simulink model "ekf_drone_3d"  (R2026a)
settings: Solver=ode4  FixedStep=0.01
libraries: simulink x1
settings Model: Creator=jaivi  LastModifiedBy=jaivi

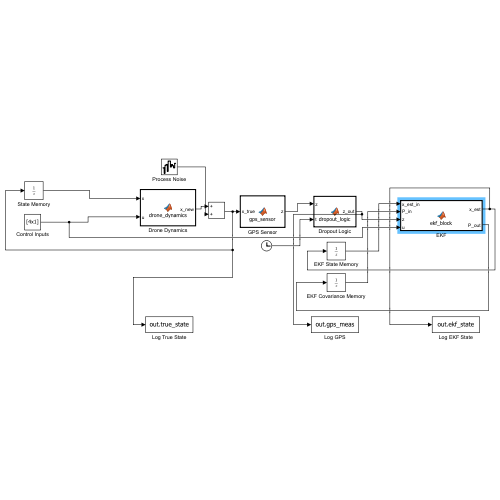
[thumbnail: Simulink's stored preview of the top-level diagram]
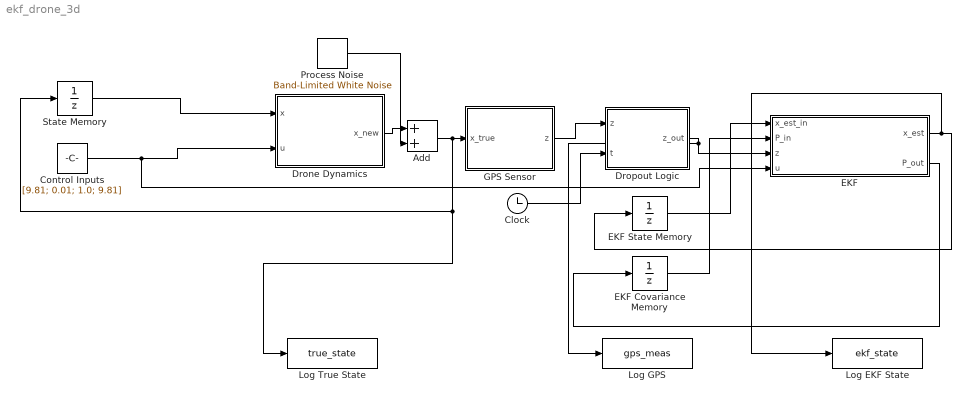
== system ekf_drone_3d ==
  Add : Sum
  Clock : Clock
  Control Inputs : Constant  Value=[9.81; 0.01; 1.0; 9.81]  OutDataTypeStr=double
  Drone Dynamics : MATLAB Function  TreatAsAtomicUnit=on
  Dropout Logic : MATLAB Function  TreatAsAtomicUnit=on
  EKF : MATLAB Function  TreatAsAtomicUnit=on
  EKF Covariance Memory : UnitDelay  InitialCondition=0.1*ones(64,1)  SampleTime=0.01
  EKF State Memory : UnitDelay  InitialCondition=[0; 0; 10; 0; 0; 0; 0; 0]  SampleTime=0.01
  GPS Sensor : MATLAB Function  TreatAsAtomicUnit=on
  Log EKF State : ToWorkspace  VariableName=ekf_state  SampleTime=-1
  Log GPS : ToWorkspace  VariableName=gps_meas  SampleTime=-1
  Log True State : ToWorkspace  VariableName=true_state  SampleTime=-1
  Process Noise : simulink/Sources/Band-Limited White Noise  Cov=[0.001 0.001 0.001 0.002 0.002 0.002 0.0001 0.0001]  Ts=0.01  seed=[23341]
  State Memory : UnitDelay  InitialCondition=[0; 0; 10; 0; 0; 0; 0; 0]  SampleTime=0.01
  wires:
  Control Inputs/1 -> EKF/4(u), Drone Dynamics/2(u)
  State Memory/1 -> Drone Dynamics/1(x)
  GPS Sensor/1(z) -> Dropout Logic/1(z)
  Clock/1 -> Dropout Logic/2(t)
  EKF State Memory/1 -> EKF/1(x_est_in)
  EKF Covariance Memory/1 -> EKF/2(P_in)
  Dropout Logic/1(z_out) -> Log GPS/1, EKF/3(z)
  EKF/1(x_est) -> Log EKF State/1, EKF State Memory/1
  EKF/2(P_out) -> EKF Covariance Memory/1
  Drone Dynamics/1(x_new) -> Add/1
  Process Noise/1 -> Add/2
  Add/1 -> State Memory/1, Log True State/1, GPS Sensor/1(x_true)

== matlab function ekf_drone_3d/GPS Sensor ==
  data: x_true input; z output
function z = gps_sensor(x_true)
% GPS sensor — measures position only with noise
% x_true = [px, py, pz, vx, vy, vz, theta, phi] (8x1)
% z = [px_meas, py_meas, pz_meas] (3x1)

% Extract true position
px = x_true(1);
py = x_true(2);
pz = x_true(3);

% Add Gaussian noise (2m standard deviation)
noise = 2.0 * randn(3,1);

z = [px; py; pz] + noise;

== matlab function ekf_drone_3d/Drone Dynamics ==
  data: x input; u input; x_new output
function x_new = drone_dynamics(x, u)
% 3D drone state transition
% x = [px, py, pz, vx, vy, vz, theta, phi] (8x1)
% u = [T, dt, m, g] inputs and constants

px    = x(1);
py    = x(2);
pz    = x(3);
vx    = x(4);
vy    = x(5);
vz    = x(6);
theta = x(7);
phi   = x(8);

T  = u(1);
dt = u(2);
m  = u(3);
g  = u(4);

% Accelerations
ax =  (T/m) * sin(theta);
ay = -(T/m) * sin(phi) * cos(theta);
az =  (T/m) * cos(phi) * cos(theta) - g;

% Next state
x_new = [
    px + vx*dt;
    py + vy*dt;
    pz + vz*dt;
    vx + ax*dt;
    vy + ay*dt;
    vz + az*dt;
    theta;
    phi
];

== matlab function ekf_drone_3d/Dropout Logic ==
  data: z input; z_out output; t input
function z_out = dropout_logic(z, t)
% Cut GPS signal between t=3s and t=5s
% z = GPS measurement (3x1)
% t = current simulation time

if t >= 3.0 && t <= 5.0
    z_out = [0; 0; 0];  % no signal during dropout
else
    z_out = z;           % normal GPS signal
end

== matlab function ekf_drone_3d/EKF ==
  data: x_est_in input; P_in input; z input; u input; x_est output; P_out output
function [x_est, P_out] = ekf_block(x_est_in, P_in, z, u)
% 3D EKF block
% x_est_in = previous state estimate (8x1)
% P_in     = previous covariance (64x1, reshaped from 8x8)
% z        = GPS measurement (3x1)
% u        = control inputs [T, dt, m, g] (4x1)

% Unpack constants
T  = u(1);
dt = u(2);
m  = u(3);
g  = u(4);

% Reshape P from vector to matrix
P = reshape(P_in, 8, 8);

% Unpack state
px    = x_est_in(1);
py    = x_est_in(2);
pz    = x_est_in(3);
vx    = x_est_in(4);
vy    = x_est_in(5);
vz    = x_est_in(6);
theta = x_est_in(7);
phi   = x_est_in(8);

% Measurement matrix — GPS measures position only
H = [1 0 0 0 0 0 0 0;
     0 1 0 0 0 0 0 0;
     0 0 1 0 0 0 0 0];

% Process noise
Q = diag([0.001, 0.001, 0.001, 0.002, 0.002, 0.002, 0.0001, 0.0001]);

% Measurement noise
R = diag([2.0, 2.0, 2.0]);

% PREDICT
% State transition
ax =  (T/m) * sin(theta);
ay = -(T/m) * sin(phi) * cos(theta);
az =  (T/m) * cos(phi) * cos(theta) - g;

x_pred = [
    px + vx*dt;
    py + vy*dt;
    pz + vz*dt;
    vx + ax*dt;
    vy + ay*dt;
    vz + az*dt;
    theta;
    phi
];

% Jacobian F
F = [1  0  0  dt  0   0   0                                    0;
     0  1  0  0   dt  0   0                                    0;
     0  0  1  0   0   dt  0                                    0;
     0  0  0  1   0   0   (T/m)*cos(theta)*dt                  0;
     0  0  0  0   1   0   (T/m)*sin(phi)*sin(theta)*dt        -(T/m)*cos(phi)*cos(theta)*dt;
     0  0  0  0   0   1  -(T/m)*cos(phi)*sin(theta)*dt        -(T/m)*sin(phi)*cos(theta)*dt;
     0  0  0  0   0   0   1                                    0;
     0  0  0  0   0   0   0                                    1];

P_pred = F * P * F' + Q;

% CHECK FOR GPS DROPOUT
% If z is all zeros, skip update step
if norm(z) < 0.001
    % Dropout — predict only
    x_est  = x_pred;
    P_out  = reshape(P_pred, 64, 1);
else
    % UPDATE
    y = z - H * x_pred;
    S = H * P_pred * H' + R;
    K = P_pred * H' / S;
    x_est = x_pred + K * y;
    P_new = (eye(8) - K*H) * P_pred;
    P_out = reshape(P_new, 64, 1);
end
